simulink model "sendex"  (R2020b)
settings: Solver=FixedStepAuto  StartTime=0.0  StopTime=inf  FixedStep=0.001  RelTol=1e-3
undefined symbols (not defined in the file): autopilot, control, kspTxIn0
libraries: ksplib x1
settings Model: EnablePacing=on  Creator=brianhannan  LastModifiedBy=brianhannan

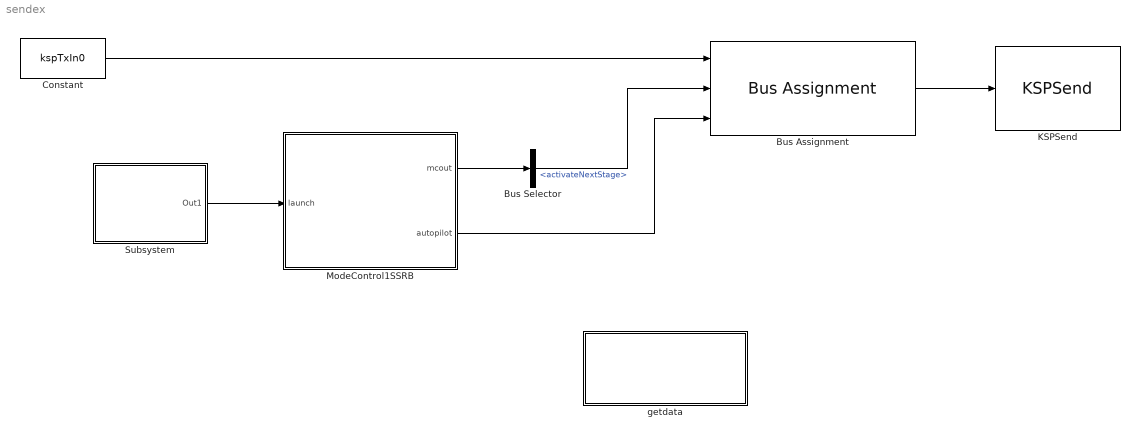
== system sendex ==
  Bus Assignment : BusAssignment  AssignedSignals=control.activateNextStage,autopilot
  Bus Selector : BusSelector  OutputSignals=activateNextStage
  Constant : Constant  Value=kspTxIn0  OutDataTypeStr=Bus: kspTxIn
  KSPSend : ksplib/KSPSend  SimulateUsing=Interpreted execution
  ModeControl1SSRB : Stateflow chart  TreatAsAtomicUnit=on  mask(ModeControl){apPitch=90, apHeading=90}
      mask prompts: apPitch "Autopilot pitch:"; apHeading "Autopilot heading:"
      mask help: Mode control
  Subsystem : Subsystem  mask{tLaunch=3}
      mask prompts: tLaunch "Launch time:"
      mask Display: disp('Launch command');
  getdata : Subsystem
      settings: OpenFcn=setupLaunchExample;
      mask Display: disp('get model data')
  wires:
  Constant/1 -> Bus Assignment/1
  Bus Assignment/1 -> KSPSend/1
  ModeControl1SSRB/1(mcout) -> Bus Selector/1
  Bus Selector/1 -> Bus Assignment/2  "<activateNextStage>"
  ModeControl1SSRB/2(autopilot) -> Bus Assignment/3
  Subsystem/1(Out1) -> ModeControl1SSRB/1(launch)

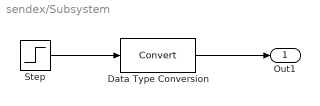
== system sendex/Subsystem ==
  Data Type Conversion : DataTypeConversion
  Step : Step  Time=tLaunch  SampleTime=0
  Out1 : Outport
  wires:
  Data Type Conversion/1 -> Out1/1
  Step/1 -> Data Type Conversion/1

== system sendex/getdata ==

== stateflow chart sendex/ModeControl1SSRB ==
  state Prelaunch
    en:
    mcout.mode = int8(-100);
    autopilot.targetPitch = apPitch;
    autopilot.targetHeading = apHeading;
    autopilot.engage = true;
  state Launch
    en:
    mcout.mode = int8(0);
    state PreFlightChecks
      en:
      % to do: add prelaunch check logic
      launchChecksOK = true;
    (default) -> PreFlightChecks
  state Ascent
    en:
    mcout.mode = int8(100);
    du:
    if ~launchCmdSent
    after(1,sec);
    mcout.activateNextStage = true;
    launchCmdSent = true;
    else
    mcout.activateNextStage = false;
    end
  state Stage1Separation
    en:
    mcout.mode = int8(200);
    du:
    if ~stage1sepCmdSent
    mcout.activateNextStage = true;
    stage1sepCmdSent = true;
    else
    mcout.activateNextStage = false;
    end
  (default) -> Prelaunch
  Prelaunch -> Launch : [launch == true]
  Launch -> (junction 31) [order 1] : [launchChecksOK == true]
  (junction 31) -> Ascent : [after(0.5,sec)]
  Ascent -> (junction 27)
  (junction 27) -> Stage1Separation [order 1] : [t>125]
  (junction 27) -> (junction 29) [order 2]
  Launch -> Prelaunch [order 2] : [launchChecksOK == false]
  data: launch input boolean size=1; mcout output Bus: mcout size=1; launchChecksOK local boolean =true; autopilot output Bus: autopilot; apPitch parameter size=1; apHeading parameter size=1; launchCmdSent local boolean =false; stage1sepCmdSent local boolean =false
